simulink model "indMotorSpeedControl2"  (R2023b)
settings: Solver=VariableStepAuto  StartTime=0.0  StopTime=30  RelTol=1e-3
libraries: spsMosfetLib x6, simulink x4, spsAsynchronousMachineSIUnitsLib x1, spsDCVoltageSourceLib x1, spsGroundLib x1, spsThreePhaseVIMeasurementLib x1, sps_lib x1
settings Model: Creator=klysm  LastModifiedBy=klysm

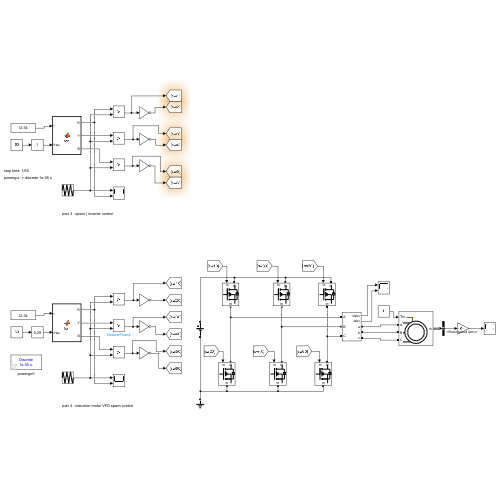
[thumbnail: Simulink's stored preview of the top-level diagram]
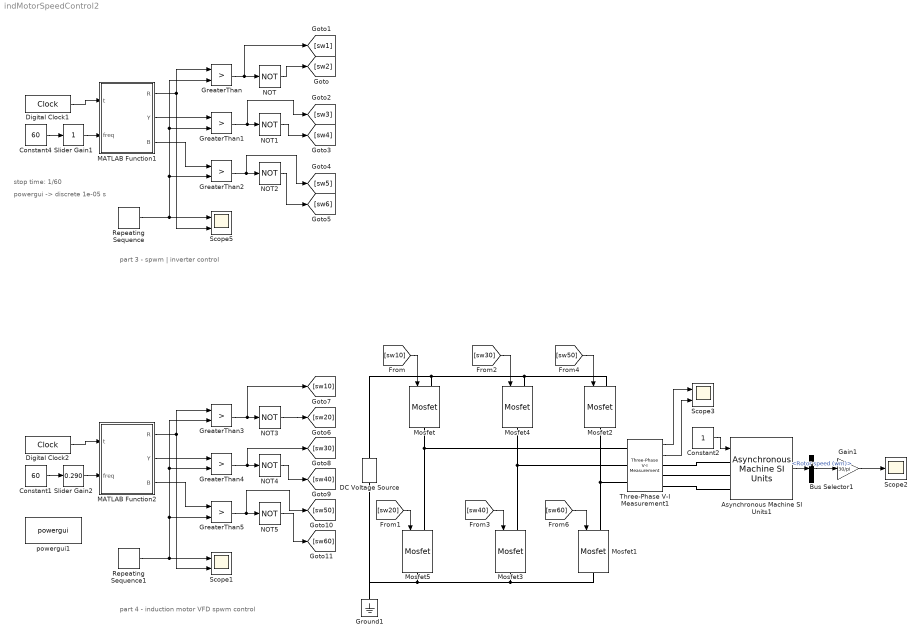
== system indMotorSpeedControl2 ==
  note: powergui -> discrete 1e-05 s
  note: stop time: 1/60
  note: part 3 - spwm | inverter control
  note: part 4 - induction motor VFD spwm control
  Asynchronous Machine SI Units1 : spsAsynchronousMachineSIUnitsLib/Asynchronous Machine SI Units  RotorType=Squirrel-cage  PresetModel="14:  200 HP 575 V 60Hz 1785 RPM"  MechanicalLoad=Torque Tm  ShowDetailedParameters=on  ReferenceFrame=Rotor  Units=SI  MeasurementBus=off  NominalParameters=[1.492e+05 575 60]  VoltageRatio=1  Stator=[0.02475 0.000284]  Rotor=[0.01329 0.000284]  Cage1=[0.4155 0.002066]  Cage2=[0.4168 0.0003495]  Lm=0.01425  Mechanical=[2.6 0.06346 2]  PolePairs=2  InitialConditions=[0 0 0 0 0 0 0 0]  SimulateSaturation=off  Saturation=[14.03593122, 27.81365428, 53.79336849, 72.68890987, 97.98006896, 148.6815601, 215.7428561, 302.9841135, 428.7778367 ; 230, 322, 414, 460, 506, 552, 598, 644, 690]  LoadFlowParameters=1492000  TsPowergui=0  TsBlock=-1  IterativeModel=Trapezoidal non iterative  IterativeDiscreteModel=Trapezoidal non iterative  Pmec=1.492e+006
  Bus Selector1 : BusSelector  OutputSignals=Mechanical.Rotor speed (wm)
  Constant1 : Constant  Value=60
  Constant2 : Constant
  Constant4 : Constant  Value=60
  DC Voltage Source : spsDCVoltageSourceLib/DC Voltage Source  Amplitude=575  Measurements=None
  Digital Clock1 : DigitalClock  SampleTime=1e-5
  Digital Clock2 : DigitalClock  SampleTime=1e-5
  Gain1 : Gain  Gain=30/pi
  GreaterThan{,1..5} (6 alike) : RelationalOperator  Operator=>  OutDataTypeStr=boolean  RndMeth=Simplest  InputSameDT=off
  Ground1 : spsGroundLib/Ground  LConnTagsString=a
  MATLAB Function1 : MATLAB Function  TreatAsAtomicUnit=on
  MATLAB Function2 : MATLAB Function  TreatAsAtomicUnit=on
  Mosfet{,1..5} (6 alike) : spsMosfetLib/Mosfet  Ron=0.1  Lon=0  Rd=0.01  Vfd=0  IC=0  Rs=1e5  Cs=inf  Measurements=off
  NOT{,1..5} (6 alike) : Logic  Operator=NOT  IconShape=distinctive  AllPortsSameDT=off  OutDataTypeStr=boolean
  Repeating Sequence : simulink/Sources/Repeating Sequence  rep_seq_t=[0 .25 .50 .75 1]*1/5000  rep_seq_y=[0 1 0 -1 0]
  Repeating Sequence1 : simulink/Sources/Repeating Sequence  rep_seq_t=[0 .25 .50 .75 1]*1/5000  rep_seq_y=[0 1 0 -1 0]
  Scope1 : Scope  NumInputPorts=2
  Scope2 : Scope
  Scope3 : Scope  NumInputPorts=2
  Scope5 : Scope  NumInputPorts=2
  Slider Gain1 : simulink/Math Operations/Slider Gain  gain=1  low=0  high=1
  Slider Gain2 : simulink/Math Operations/Slider Gain  gain=0.290  low=0  high=1
  Three-Phase V-I Measurement1 : spsThreePhaseVIMeasurementLib/Three-Phase V-I Measurement  VoltageMeasurement=phase-to-ground  SetLabelV=off  LabelV=Vabc  Vpu=off  VpuLL=off  CurrentMeasurement=yes  SetLabelI=off  LabelI=Iabc  Ipu=off  Pbase=100e6  Vbase=500e3  OutputType=Complex  PhasorSimulation=off  PSBequivalent=0
  powergui1 : sps_lib/powergui  Priority=1  SimulationMode=Discrete  SampleTime=1e-5  frequency=60  Iterations=50  frequencyindice=60  Pbase=100e6  ErrMax=1e-4  UnitsV=kV  UnitsW=MW  buscounter=0  FunctionMessages=off  echomessages=off  EnableUseOfTLC=off  CurrentSourceSwitches=off  DisableSnubberDevices=off  DisableRonSwitches=off  DisableVfSwitches=off  DisplayEquations=off  AutomaticDiscreteSolvers=off  SolverType=Tustin/Backward Euler (TBE)  Interpol=off  ExternalGateDelay=off  methode=off  Ts=100  x0status=blocks  SPID=on  SwTol=0  HookPort=off  NonlinearTolerance=1e-4  nMaxIteration=100  ContinueOnMaxIteration=off  RestoreLinks=warning  ResistiveCurrentMeasurement=off  Frange=[0:2:500]  Ylog=off  Xlog=on  ShowGrid=off  save=off  variable=ZData  structure=0  ZoomFFT=off  StartTime=0.0  cycles=1  DisplayStyle=1  fundamental=60  FreqAxis=off  MaxFrequency=1000  frequencyindicesteady=1  RmsSteady=1  display=off
  wires:
  NOT1/1 -> [sw4]
  NOT2/1 -> [sw6]
  GreaterThan2/1 -> [sw5], NOT2/1
  NOT/1 -> [sw2]
  GreaterThan1/1 -> [sw3], NOT1/1
  Repeating Sequence/1 -> GreaterThan/2, GreaterThan1/2, GreaterThan2/2, Scope5/1
  MATLAB Function1/2(Y) -> GreaterThan1/1
  MATLAB Function1/3(B) -> GreaterThan2/1
  Digital Clock1/1 -> MATLAB Function1/1(t)
  Slider Gain1/1 -> MATLAB Function1/2(freq)
  MATLAB Function1/1(R) -> GreaterThan/1, Scope5/2
  Constant4/1 -> Slider Gain1/1
  NOT4/1 -> [sw40]
  NOT3/1 -> [sw20]
  GreaterThan4/1 -> [sw30], NOT4/1
  NOT5/1 -> [sw60]
  GreaterThan3/1 -> [sw10], NOT3/1
  GreaterThan5/1 -> [sw50], NOT5/1
  Constant1/1 -> Slider Gain2/1
  MATLAB Function2/1(R) -> GreaterThan3/1, Scope1/2
  Slider Gain2/1 -> MATLAB Function2/2(freq)
  Digital Clock2/1 -> MATLAB Function2/1(t)
  Repeating Sequence1/1 -> GreaterThan3/2, GreaterThan4/2, GreaterThan5/2, Scope1/1
  MATLAB Function2/3(B) -> GreaterThan5/1
  MATLAB Function2/2(Y) -> GreaterThan4/1
  GreaterThan/1 -> [sw1], NOT/1
  [sw50] -> Mosfet2/1
  [sw30] -> Mosfet4/1
  [sw10] -> Mosfet/1
  [sw20] -> Mosfet5/1
  [sw40] -> Mosfet3/1
  [sw60] -> Mosfet1/1
  Three-Phase V-I Measurement1/1 -> Scope3/1
  Gain1/1 -> Scope2/1
  Three-Phase V-I Measurement1/2 -> Scope3/2
  Bus Selector1/1 -> Gain1/1  "<Rotor speed (wm)>"
  Asynchronous Machine SI Units1/1 -> Bus Selector1/1
  Constant2/1 -> Asynchronous Machine SI Units1/1
  connections:
  Mosfet/LConn1 -- DC Voltage Source/RConn1 -- Mosfet2/LConn1 -- Mosfet4/LConn1
  Mosfet/RConn1 -- Mosfet5/LConn1 -- Three-Phase V-I Measurement1/LConn1
  Mosfet5/RConn1 -- Ground1/LConn1 -- DC Voltage Source/LConn1 -- Mosfet1/RConn1 -- Mosfet3/RConn1
  Mosfet3/LConn1 -- Three-Phase V-I Measurement1/LConn2 -- Mosfet4/RConn1
  Mosfet1/LConn1 -- Three-Phase V-I Measurement1/LConn3 -- Mosfet2/RConn1
  Three-Phase V-I Measurement1/RConn2 -- Asynchronous Machine SI Units1/LConn2
  Three-Phase V-I Measurement1/RConn1 -- Asynchronous Machine SI Units1/LConn1
  Three-Phase V-I Measurement1/RConn3 -- Asynchronous Machine SI Units1/LConn3

== matlab function indMotorSpeedControl2/MATLAB Function1 ==
  data: t input; R output; freq input; Y output; B output
function [R,Y,B] = fcn(t,freq)
omega=2*pi*freq;
R=sin(omega*t)*freq/60;
Y=sin(omega*t+120*pi/180)*freq/60;
B=sin(omega*t+240*pi/180)*freq/60;

== matlab function indMotorSpeedControl2/MATLAB Function2 ==
  data: t input; R output; freq input; Y output; B output
function [R,Y,B] = fcn(t,freq)
omega=2*pi*freq;
R=sin(omega*t)*freq/60;
B=sin(omega*t+120*pi/180)*freq/60;
Y=sin(omega*t+240*pi/180)*freq/60;
